simulink model "mdatastore"  (Simulink 6.3)
settings: Solver=ode3  StartTime=0.0  StopTime=10.0  RelTol=1e-3
settings Model: Creator=mshakeri  LastModifiedBy=mshakeri  ExtModeAutoUpdateStatusClock=off  StrictBusMsg=ErrorLevel1
settings OptimizationCC: InlineParams=on

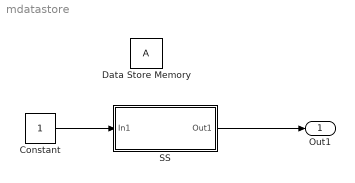
== system mdatastore ==
  Constant : Constant  SampleTime=1
  Data Store Memory : DataStoreMemory  DataStoreName=A  ReadBeforeWriteMsg=warning  WriteAfterWriteMsg=warning  WriteAfterReadMsg=warning  InitialValue=0
  SS : Subsystem  TreatAsAtomicUnit=on
  Out1 : Outport
  wires:
  Constant/1 -> SS/1(In1)
  SS/1(Out1) -> Out1/1

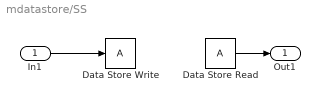
== system mdatastore/SS ==
  In1 : Inport  Port=1  LatchInput=off
  Data Store Read : DataStoreRead  DataStoreName=A  SampleTime=0
  Data Store Write : DataStoreWrite  DataStoreName=A  SampleTime=-1
  Out1 : Outport
  wires:
  In1/1 -> Data Store Write/1
  Data Store Read/1 -> Out1/1
